simulink model "Model"  (R2022b)
settings: Solver=ode4  StartTime=0.0  StopTime=20  RelTol=1e-3
settings Model: Creator=mrezk  LastModifiedBy=mrezk

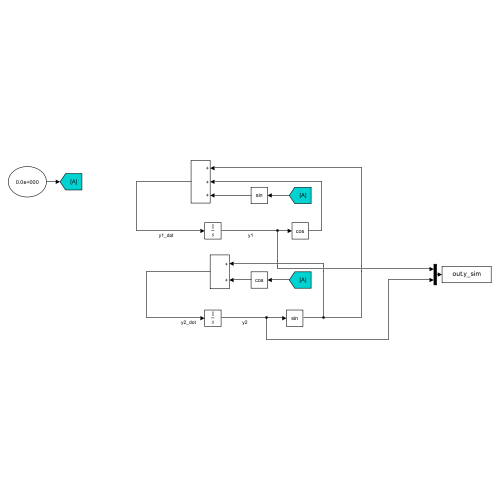
[thumbnail: Simulink's stored preview of the top-level diagram]
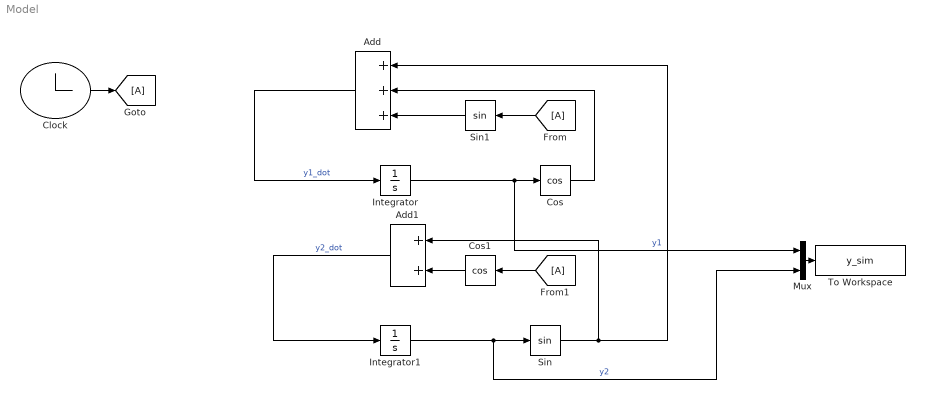
== system Model ==
  Add : Sum  Inputs=+++
  Add1 : Sum
  Clock : Clock
  Cos : Trigonometry  Operator=cos
  Cos1 : Trigonometry  Operator=cos
  From : From
  From1 : From
  Goto : Goto
  Integrator : Integrator  InitialCondition=1.3818
  Integrator1 : Integrator  InitialCondition=1.8415
  Mux : Mux  Inputs=2
  Sin : Trigonometry
  Sin1 : Trigonometry
  To Workspace : ToWorkspace  VariableName=y_sim  SampleTime=-1
  wires:
  Add/1 -> Integrator/1  "y1_dot"
  Integrator/1 -> Mux/1, Cos/1  "y1"
  Add1/1 -> Integrator1/1  "y2_dot"
  Integrator1/1 -> Mux/2, Sin/1  "y2"
  Cos/1 -> Add/2
  Sin/1 -> Add1/1, Add/1
  Clock/1 -> Goto/1
  From/1 -> Sin1/1
  Sin1/1 -> Add/3
  From1/1 -> Cos1/1
  Cos1/1 -> Add1/2
  Mux/1 -> To Workspace/1
